simulink model "ex5"  (R2014a)
settings: Solver=ode3  StartTime=0.0  StopTime=5.24288  FixedStep=2e-5  RelTol=1e-3
undefined symbols (not defined in the file or in its folder): gcbh, rcfiltgaincompat
libraries: commfilt2 x4, commchan3 x2, commrandsrc2 x2
settings Model: CovSFcnEnable=on  Creator=ctu  LastModifiedBy=akenge
settings OptimizationCC: SimCompilerOptimization=off
settings DebuggingCC: MergeDetectMultiDrivingBlocksExec=error  SolverPrmCheckMsg=none  FrameProcessingCompatibilityMsg=error
settings RTWCC: RTWCompilerOptimization=off

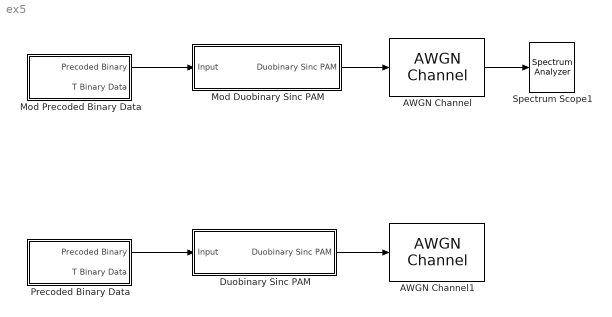
== system ex5 ==
  AWGN Channel : commchan3/AWGN Channel  InputProcessing=Inherited (this choice will be removed - see release notes)  seed=randseed  noiseMode=Variance from mask  EbNodB=10  EsNodB=10  SNRdB=10  bitsPerSym=1  Ps=1  Tsym=1  variance=10
  AWGN Channel1 : commchan3/AWGN Channel  InputProcessing=Inherited (this choice will be removed - see release notes)  seed=randseed  noiseMode=Variance from mask  EbNodB=10  EsNodB=10  SNRdB=10  bitsPerSym=1  Ps=1  Tsym=1  variance=10
  Duobinary Sinc PAM : Subsystem
  Mod Duobinary Sinc PAM : Subsystem
  Mod Precoded Binary Data : Subsystem
  Precoded Binary Data : Subsystem
  Spectrum Scope1 : SpectrumAnalyzer
  wires:
  Mod Duobinary Sinc PAM/1(Duobinary Sinc PAM) -> AWGN Channel/1
  Mod Precoded Binary Data/1(Precoded Binary) -> Mod Duobinary Sinc PAM/1(Input)
  Duobinary Sinc PAM/1(Duobinary Sinc PAM) -> AWGN Channel1/1
  Precoded Binary Data/1(Precoded Binary) -> Duobinary Sinc PAM/1(Input)
  AWGN Channel/1 -> Spectrum Scope1/1

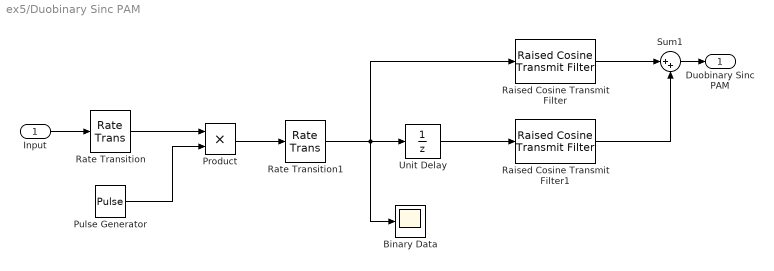
== system ex5/Duobinary Sinc PAM ==
  Input : Inport
  Binary Data : Scope
      settings: YMin=-1.5  YMax=1.5  SaveName=ScopeData2
  Product : Product
  Pulse Generator : DiscretePulseGenerator  PulseType=Time based  Period=1e-3  PulseWidth=2
  Raised Cosine Transmit Filter : commfilt2/Raised Cosine Transmit Filter  filtType=Normal  filtSpan=2*((8)/2)  currentFiltSpan=2*((8)/2)  D=(8)/2  R=0  sampMode=Mute  saveAsFlag=0  N=50  framing=Allow multirate processing  InputProcessing=Inherited (this choice will be removed - see release notes)  checkGain=Normalized  filterGain=rcfiltgaincompat(gcbh)  checkCoeff=off  variableName=rcTxFilt  launchFVT=on  roundingMode=Floor  overflowMode=off
  Raised Cosine Transmit Filter1 : commfilt2/Raised Cosine Transmit Filter  filtType=Normal  filtSpan=2*((8)/2)  currentFiltSpan=2*((8)/2)  D=(8)/2  R=0  sampMode=Mute  saveAsFlag=0  N=50  framing=Allow multirate processing  InputProcessing=Inherited (this choice will be removed - see release notes)  checkGain=Normalized  filterGain=rcfiltgaincompat(gcbh)  checkCoeff=off  variableName=rcTxFilt1  launchFVT=on  roundingMode=Floor  overflowMode=off
  Rate Transition : RateTransition  OutPortSampleTime=2e-5
  Rate Transition1 : RateTransition  OutPortSampleTime=1e-3
  Sum1 : Sum  Inputs=|++
  Unit Delay : UnitDelay  SampleTime=-1
  Duobinary Sinc PAM : Outport
  wires:
  Rate Transition/1 -> Product/1
  Pulse Generator/1 -> Product/2
  Product/1 -> Rate Transition1/1
  Sum1/1 -> Duobinary Sinc PAM/1
  Rate Transition1/1 -> Binary Data/1, Raised Cosine Transmit Filter/1, Unit Delay/1
  Unit Delay/1 -> Raised Cosine Transmit Filter1/1
  Raised Cosine Transmit Filter1/1 -> Sum1/2
  Raised Cosine Transmit Filter/1 -> Sum1/1
  Input/1 -> Rate Transition/1

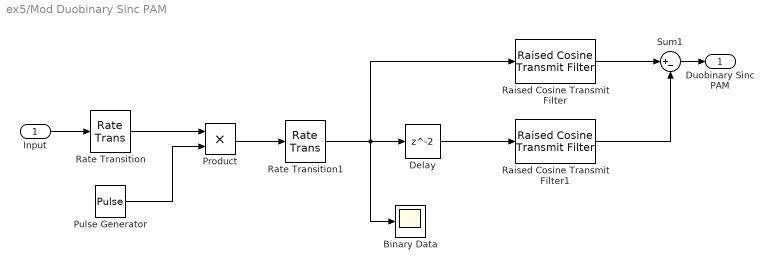
== system ex5/Mod Duobinary Sinc PAM ==
  Input : Inport
  Binary Data : Scope
      settings: YMin=-1.5  YMax=1.5  SaveName=ScopeData2
  Delay : Delay  InitialCondition=0  InputProcessing=Inherited
  Product : Product
  Pulse Generator : DiscretePulseGenerator  PulseType=Time based  Period=1e-3  PulseWidth=2
  Raised Cosine Transmit Filter : commfilt2/Raised Cosine Transmit Filter  filtType=Normal  filtSpan=8  currentFiltSpan=8  D=(8)/2  R=0  sampMode=Mute  saveAsFlag=0  N=50  framing=Allow multirate processing  InputProcessing=Inherited (this choice will be removed - see release notes)  checkGain=Normalized  filterGain=(5)*rcfiltgaincompat(gcbh)  checkCoeff=off  variableName=rcTxFilt  launchFVT=on  roundingMode=Floor  overflowMode=off
  Raised Cosine Transmit Filter1 : commfilt2/Raised Cosine Transmit Filter  filtType=Normal  filtSpan=8  currentFiltSpan=8  D=(8)/2  R=0  sampMode=Mute  saveAsFlag=0  N=50  framing=Allow multirate processing  InputProcessing=Inherited (this choice will be removed - see release notes)  checkGain=Normalized  filterGain=(5)*rcfiltgaincompat(gcbh)  checkCoeff=off  variableName=rcTxFilt1  launchFVT=on  roundingMode=Floor  overflowMode=off
  Rate Transition : RateTransition  OutPortSampleTime=2e-5
  Rate Transition1 : RateTransition  OutPortSampleTime=1e-3
  Sum1 : Sum  Inputs=|+-
  Duobinary Sinc PAM : Outport
  wires:
  Rate Transition/1 -> Product/1
  Pulse Generator/1 -> Product/2
  Product/1 -> Rate Transition1/1
  Sum1/1 -> Duobinary Sinc PAM/1
  Rate Transition1/1 -> Delay/1, Binary Data/1, Raised Cosine Transmit Filter/1
  Delay/1 -> Raised Cosine Transmit Filter1/1
  Raised Cosine Transmit Filter1/1 -> Sum1/2
  Raised Cosine Transmit Filter/1 -> Sum1/1
  Input/1 -> Rate Transition/1

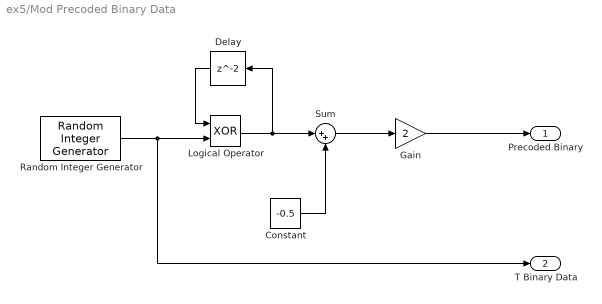
== system ex5/Mod Precoded Binary Data ==
  Constant : Constant  Value=-0.5
  Delay : Delay  InitialCondition=0  InputProcessing=Inherited
  Gain : Gain  Gain=2
  Logical Operator : Logic  Operator=XOR  AllPortsSameDT=off  OutDataTypeStr=boolean
  Random Integer Generator : commrandsrc2/Random Integer Generator  mul=2  seed=randseed  Ts=1e-3  frameBased=off  sampPerFrame=1  orient=off  outDataType=boolean
  Sum : Sum  Inputs=|++
  Precoded Binary : Outport
  T Binary Data : Outport  Port=2
  wires:
  Random Integer Generator/1 -> T Binary Data/1, Logical Operator/2
  Delay/1 -> Logical Operator/1
  Logical Operator/1 -> Delay/1, Sum/1
  Constant/1 -> Sum/2
  Sum/1 -> Gain/1
  Gain/1 -> Precoded Binary/1

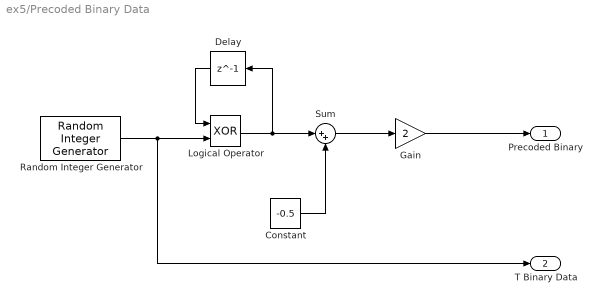
== system ex5/Precoded Binary Data ==
  Constant : Constant  Value=-0.5
  Delay : Delay  DelayLength=1  InitialCondition=0  InputProcessing=Inherited
  Gain : Gain  Gain=2
  Logical Operator : Logic  Operator=XOR  AllPortsSameDT=off  OutDataTypeStr=boolean
  Random Integer Generator : commrandsrc2/Random Integer Generator  mul=2  seed=randseed  Ts=1e-3  frameBased=off  sampPerFrame=1  orient=off  outDataType=boolean
  Sum : Sum  Inputs=|++
  Precoded Binary : Outport
  T Binary Data : Outport  Port=2
  wires:
  Random Integer Generator/1 -> T Binary Data/1, Logical Operator/2
  Delay/1 -> Logical Operator/1
  Logical Operator/1 -> Delay/1, Sum/1
  Constant/1 -> Sum/2
  Sum/1 -> Gain/1
  Gain/1 -> Precoded Binary/1
